simulink model "attitude_block"  (R2025b)
settings: Solver=FixedStepDiscrete  StartTime=0  StopTime=1.0  FixedStep=0.0012005  RelTol=1e-3
settings Model: Creator=Ashwin  LastModifiedBy=Ashwin

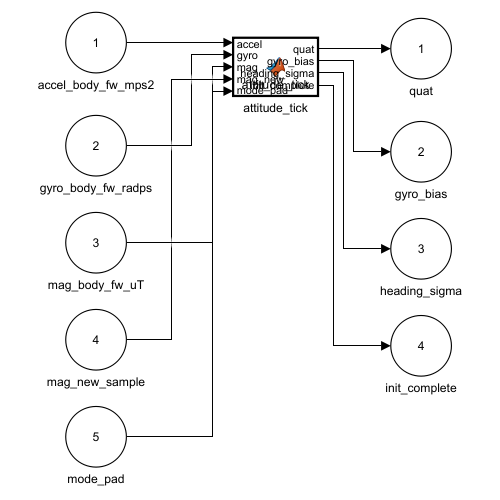
[thumbnail: Simulink's stored preview of the top-level diagram]
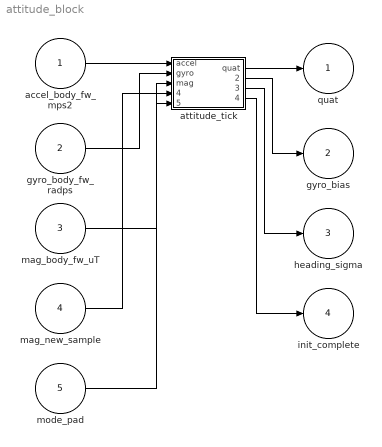
== system attitude_block ==
  accel_body_fw_mps2 : Inport  PortDimensions=3  SampleTime=0.0012005
  gyro_body_fw_radps : Inport  Port=2  PortDimensions=3  SampleTime=0.0012005
  mag_body_fw_uT : Inport  Port=3  PortDimensions=3  SampleTime=0.0012005
  mag_new_sample : Inport  Port=4  PortDimensions=1  SampleTime=0.0012005
  mode_pad : Inport  Port=5  PortDimensions=1  SampleTime=0.0012005
  attitude_tick : MATLAB Function  TreatAsAtomicUnit=on
  quat : Outport
  gyro_bias : Outport  Port=2
  heading_sigma : Outport  Port=3
  init_complete : Outport  Port=4
  wires:
  accel_body_fw_mps2/1 -> attitude_tick/1(accel)
  gyro_body_fw_radps/1 -> attitude_tick/2(gyro)
  mag_body_fw_uT/1 -> attitude_tick/3(mag)
  mag_new_sample/1 -> attitude_tick/4(mag_new)
  mode_pad/1 -> attitude_tick/5(mode_pad)
  attitude_tick/1(quat) -> quat/1
  attitude_tick/3(heading_sigma) -> heading_sigma/1
  attitude_tick/2(gyro_bias) -> gyro_bias/1
  attitude_tick/4(init_complete) -> init_complete/1

== matlab function attitude_block/attitude_tick ==
  data: accel input; quat output; gyro input; mag input; mag_new input; mode_pad input; gyro_bias output; heading_sigma output; init_complete output
function [quat, gyro_bias, heading_sigma, init_complete] = attitude_tick(accel, gyro, mag, mag_new, mode_pad)
%#codegen
    persistent st p
    if isempty(st)
        st = casper_attitude_state_new();
        % Pull params from base workspace at first call
        p = evalin('base', 'Attitude');
        if ~isfield(p, 'M_ref_nav_uT')
            p.M_ref_nav_uT = [0; 0; 50];   % default Z-up Earth field, uT
        end
    end
    [att, st] = casper_attitude_tick(accel(:), gyro(:), mag(:), logical(mag_new), logical(mode_pad), 1/833, p, st);
    quat          = att.quat_body_to_nav;
    gyro_bias     = att.gyro_bias_radps;
    heading_sigma = att.heading_sigma_rad;
    init_complete = att.init_complete;
end
